simulink model "testing_desired_rotation"  (R2024a)
settings: Solver=FixedStepAuto  StartTime=0.0  StopTime=100  FixedStep=0.01  RelTol=1e-3
libraries: sharedtransform x8, dspsigops x2
settings Model: Creator=bemran  LastModifiedBy=bemran

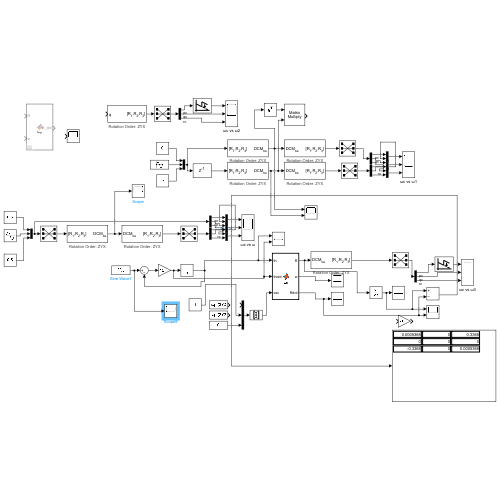
[thumbnail: Simulink's stored preview of the top-level diagram]
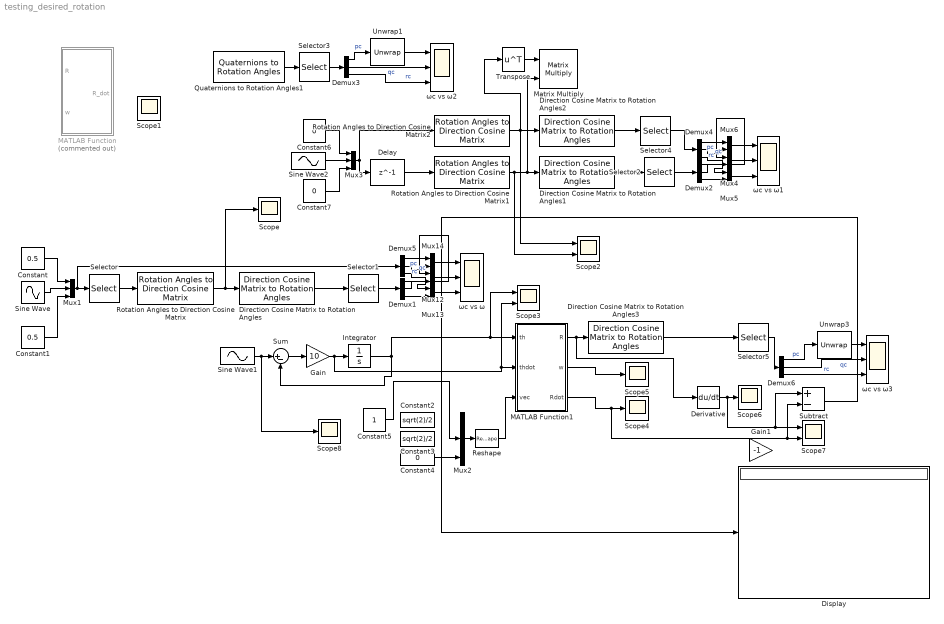
== system testing_desired_rotation ==
  Constant : Constant  Value=0.5
  Constant1 : Constant  Value=0.5
  Constant2 : Constant  Value=sqrt(2)/2
  Constant3 : Constant  Value=sqrt(2)/2
  Constant4 : Constant  Value=0
  Constant5 : Constant
  Constant6 : Constant  Value=0
  Constant7 : Constant  Value=0
  Delay : Delay  DelayLength=1  InitialCondition=[0;0;0]
  Demux{1..6} (6 alike) : Demux  Outputs=3
  Derivative : Derivative
  Direction Cosine Matrix to Rotation Angles{,1..3} (4 alike) : sharedtransform/Direction Cosine Matrix to Rotation Angles  rotationOrder=ZYX  aMode=aMode  action=None  tolerance=eps(2)
      settings: LibrarySourceBlock=|
      | aerolibtransform2/Direction Cosine Matrix
      | to Rotation Angles
  Display : Display
  Gain : Gain  Gain=10
  Gain1 : Gain  Gain=-1
  Integrator : Integrator  InitialCondition=2*pi
  MATLAB Function : MATLAB Function  Commented=on  TreatAsAtomicUnit=on
  MATLAB Function1 : MATLAB Function  TreatAsAtomicUnit=on
  Matrix Multiply : Product  Multiplication=Matrix(*)
  Mux1 : Mux  Inputs=3
  Mux{4..6,12..14} (6 alike) : Mux  Inputs=2
  Mux2 : Mux  Inputs=3
  Mux3 : Mux  Inputs=3
  Quaternions to Rotation Angles1 : sharedtransform/Quaternions to Rotation Angles  rotationOrder=ZYX  aMode=aMode
  Reshape : Reshape  OutputDimensionality=Column vector (2-D)
  Rotation Angles to Direction Cosine Matrix : sharedtransform/Rotation Angles to Direction Cosine Matrix  rotationOrder=ZYX  aMode=aMode
  Rotation Angles to Direction Cosine Matrix1 : sharedtransform/Rotation Angles to Direction Cosine Matrix  rotationOrder=ZYX  aMode=aMode
  Rotation Angles to Direction Cosine Matrix2 : sharedtransform/Rotation Angles to Direction Cosine Matrix  rotationOrder=ZYX  aMode=aMode
  Scope{,1,4..6,8} (6 alike) : Scope
  Scope2 : Scope  NumInputPorts=2
  Scope3 : Scope  NumInputPorts=2
  Scope7 : Scope  NumInputPorts=2
  Selector{,1..5} (6 alike) : Selector  InputPortWidth=3  IndexOptions=Index vector (dialog)  Indices=[3 2 1]  OutputSizes=1
  Sine Wave : Sin  Amplitude=2*pi  Frequency=0.1  SampleTime=0
  Sine Wave1 : Sin  Amplitude=2*pi  Frequency=0.1  Phase=+pi/2  SampleTime=0
  Sine Wave2 : Sin  Amplitude=2*pi  Frequency=0.1  Phase=+pi/2  SampleTime=0
  Subtract : Sum  Inputs=+-
  Sum : Sum  Inputs=|+-
  Transpose : Math  Operator=transpose
  Unwrap1 : dspsigops/Unwrap  tol=pi  InputProcessing=Columns as channels (frame based)  running=off
  Unwrap3 : dspsigops/Unwrap  tol=pi  InputProcessing=Columns as channels (frame based)  running=off
  ωc vs ω{,1..3} (4 alike) : Scope  NumInputPorts=3
  wires:
  Demux1/3 -> Mux13/2
  Mux12/1 -> ωc vs ω/2
  Demux5/1 -> Mux14/1  "pc"
  Selector1/1 -> Demux1/1
  Mux1/1 -> Demux5/1, Selector/1
  Demux5/2 -> Mux12/1  "qc"
  Demux5/3 -> Mux13/1  "rc"
  Demux1/2 -> Mux12/2
  Mux13/1 -> ωc vs ω/3
  Mux14/1 -> ωc vs ω/1
  Demux1/1 -> Mux14/2
  Constant1/1 -> Mux1/3
  Sine Wave/1 -> Mux1/2
  Constant/1 -> Mux1/1
  Selector/1 -> Rotation Angles to Direction Cosine Matrix/1
  Direction Cosine Matrix to Rotation Angles/1 -> Selector1/1
  Rotation Angles to Direction Cosine Matrix/1 -> Scope/1, Direction Cosine Matrix to Rotation Angles/1
  Constant5/1 -> Mux2/2
  Constant4/1 -> Mux2/3
  Sine Wave1/1 -> Scope8/1, Sum/1
  Unwrap1/1 -> ωc vs ω2/1
  Selector3/1 -> Demux3/1
  Demux3/3 -> ωc vs ω2/3  "rc"
  Demux3/1 -> Unwrap1/1  "pc"
  Demux3/2 -> ωc vs ω2/2  "qc"
  Quaternions to Rotation Angles1/1 -> Selector3/1
  Constant6/1 -> Mux3/1
  Sine Wave2/1 -> Mux3/2
  Constant7/1 -> Mux3/3
  Mux3/1 -> Delay/1, Rotation Angles to Direction Cosine Matrix2/1
  Rotation Angles to Direction Cosine Matrix1/1 -> Scope2/2, Matrix Multiply/2, Direction Cosine Matrix to Rotation Angles1/1
  Direction Cosine Matrix to Rotation Angles1/1 -> Selector2/1
  Demux2/1 -> Mux6/2
  Mux6/1 -> ωc vs ω1/1
  Mux5/1 -> ωc vs ω1/3
  Demux2/2 -> Mux4/2
  Demux4/3 -> Mux5/1  "rc"
  Demux4/2 -> Mux4/1  "qc"
  Selector2/1 -> Demux2/1
  Demux4/1 -> Mux6/1  "pc"
  Mux4/1 -> ωc vs ω1/2
  Demux2/3 -> Mux5/2
  Delay/1 -> Rotation Angles to Direction Cosine Matrix1/1
  Direction Cosine Matrix to Rotation Angles2/1 -> Selector4/1
  Selector4/1 -> Demux4/1
  Rotation Angles to Direction Cosine Matrix2/1 -> Transpose/1, Scope2/1, Direction Cosine Matrix to Rotation Angles2/1
  Transpose/1 -> Matrix Multiply/1
  Integrator/1 -> Scope3/1, MATLAB Function1/1(th), Sum/2
  Sum/1 -> Gain/1
  Gain/1 -> Scope3/2, MATLAB Function1/2(thdot), Integrator/1
  Mux2/1 -> Reshape/1
  Reshape/1 -> MATLAB Function1/3(vec)
  MATLAB Function1/1(R) -> Derivative/1, Direction Cosine Matrix to Rotation Angles3/1
  Selector5/1 -> Demux6/1
  Demux6/2 -> ωc vs ω3/2  "qc"
  Demux6/1 -> Unwrap3/1  "pc"
  Demux6/3 -> ωc vs ω3/3  "rc"
  MATLAB Function1/3(Rdot) -> Subtract/2, Scope7/2, Scope4/1
  MATLAB Function1/2(w) -> Scope5/1
  Direction Cosine Matrix to Rotation Angles3/1 -> Selector5/1
  Unwrap3/1 -> ωc vs ω3/1
  Derivative/1 -> Subtract/1, Scope7/1, Scope6/1
  Subtract/1 -> Display/1

== matlab function testing_desired_rotation/MATLAB Function1 ==
  data: R output size=[3 3]; th input size=[1]; thdot input size=[1]; vec input; w output size=[3 1]; Rdot output size=[3 3]
function [R, w, Rdot]  = fcn(th, thdot, vec)
R = eye(3) * sin(th) * Skew(vec) + (1-cos(th))*(vec*vec'-eye(3));
w = thdot * vec;
Rdot = R * Skew(w);

function mat = Skew(vec)
    mat = [      0, -vec(3),  vec(2);...
            vec(3),       0, -vec(1);...
           -vec(2),  vec(1),     0];
end
end

== matlab function testing_desired_rotation/MATLAB Function ==
  data: R_dot output size=[3 3]; R input size=[3 3]; w input size=[3 1]
function R_dot  = fcn(R, w)
R_dot = R * Skew(w);

function Mat = Skew(vec)
    mat = [      0, -vec(3),  vec(2);...
            vec(3),       0, -vec(1);...
           -vec(2),  vec(1),     0];
end
end
